simulink model "pool_task"  (Simulink 3.00)
libraries: mathlib x13, logiclib x10, execlib x2, genlib x1, timelib x1

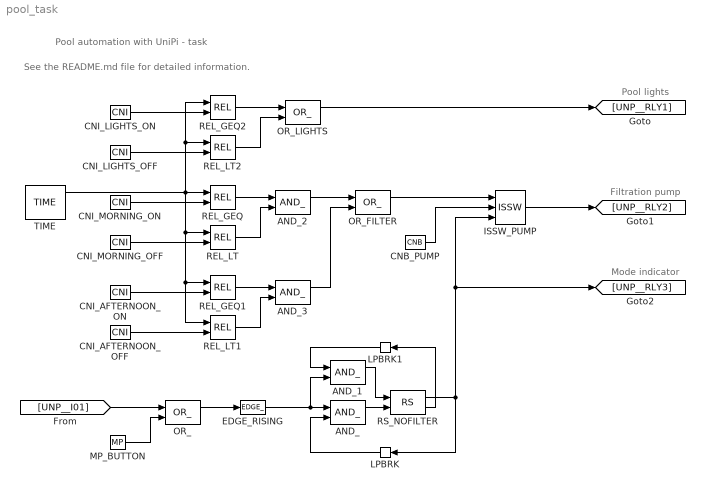
== system pool_task ==
  note: Pool lights
  note: Filtration pump
  note: Mode indicator
  note: See the README.md file for detailed information.
  note: Pool automation with UniPi - task
  AND_{,1..3} (4 alike) : logiclib/AND_
  CNB_PUMP : mathlib/CNB  YCN=off
  CNI_AFTERNOON_OFF : mathlib/CNI  icn=14
  CNI_AFTERNOON_ON : mathlib/CNI  icn=13
  CNI_LIGHTS_OFF : mathlib/CNI  icn=1
  CNI_LIGHTS_ON : mathlib/CNI  icn=21
  CNI_MORNING_OFF : mathlib/CNI  icn=4
  CNI_MORNING_ON : mathlib/CNI  icn=2
  EDGE_RISING : logiclib/EDGE_  iedge=1: Rising edge
  ISSW_PUMP : logiclib/ISSW
  LPBRK : execlib/LPBRK  Orientation=left
  LPBRK1 : execlib/LPBRK  Orientation=left
  MP_BUTTON : genlib/MP  pwidth=1  BSTATE=off  RPTF=off
  OR_ : logiclib/OR_
  OR_FILTER : logiclib/OR_
  OR_LIGHTS : logiclib/OR_
  REL_GEQ : mathlib/REL  irel=6: greater or equal (>=)
  REL_GEQ1 : mathlib/REL  irel=6: greater or equal (>=)
  REL_GEQ2 : mathlib/REL  irel=6: greater or equal (>=)
  REL_LT : mathlib/REL  irel=3: less than (<)
  REL_LT1 : mathlib/REL  irel=3: less than (<)
  REL_LT2 : mathlib/REL  irel=3: less than (<)
  RS_NOFILTER : logiclib/RS
  TIME : timelib/TIME  tz=1: Local time
  wires:
  AND_/1 -> RS_NOFILTER/2
  AND_1/1 -> RS_NOFILTER/1
  AND_2/1 -> OR_FILTER/1
  AND_3/1 -> OR_FILTER/2
  CNB_PUMP/1 -> ISSW_PUMP/2
  CNI_AFTERNOON_OFF/1 -> REL_LT1/2
  CNI_AFTERNOON_ON/1 -> REL_GEQ1/2
  CNI_LIGHTS_OFF/1 -> REL_LT2/2
  CNI_LIGHTS_ON/1 -> REL_GEQ2/2
  CNI_MORNING_OFF/1 -> REL_LT/2
  CNI_MORNING_ON/1 -> REL_GEQ/2
  EDGE_RISING/1 -> AND_/1, AND_1/2
  [UNP__I01] -> OR_/1
  ISSW_PUMP/1 -> [UNP__RLY2]
  LPBRK/1 -> AND_/2
  LPBRK1/1 -> AND_1/1
  MP_BUTTON/1 -> OR_/2
  OR_/1 -> EDGE_RISING/1
  OR_FILTER/1 -> ISSW_PUMP/1
  OR_LIGHTS/1 -> [UNP__RLY1]
  REL_GEQ/1 -> AND_2/1
  REL_GEQ1/1 -> AND_3/1
  REL_GEQ2/1 -> OR_LIGHTS/1
  REL_LT/1 -> AND_2/2
  REL_LT1/1 -> AND_3/2
  REL_LT2/1 -> OR_LIGHTS/2
  RS_NOFILTER/1 -> LPBRK/1, [UNP__RLY3], ISSW_PUMP/3
  RS_NOFILTER/2 -> LPBRK1/1
  TIME/1 -> REL_GEQ/1, REL_LT/1, REL_GEQ1/1, REL_LT1/1, REL_GEQ2/1, REL_LT2/1
